simulink model "sim_impcont"  (R2016a)
settings: Solver=ode23tb  StartTime=0.0  StopTime=t(end)  MaxStep=1e-3
InitFcn:
  | fp_k=12000;
  | fp_d=10*2e2;
  | w=11;
  | stiff=0.1;
  | damp=1;
values from neighbouring files (symbols this model uses):
  N = length(shin_angles_in.signals.values)    [GaitEmu_code.m]    (also in dy1.m; dy2.m; est_joint.m = size( [body1.trans body2.trans], 1 ); impcont.m)
  s = [-atan((t2.*3.379e-4+t3+t4.*t5.*4.401e-2)./(t4.*cos(q2)));-asin(t2.*1.4870979e-5+t3.*4.401e-2-t4.*t5)]    [FK_af.m]    (also in FK_footimp.m = [atan((ree2_1.*t2.*4.401e-2+ree2_2.*t4+ree2_3.*t3+t5.*t7.*4.; FK_gaitEmul.m = [q1+t2.*t4.*4.234e-1+t3.*t5.*1.5e-3-t2.*t6.*t7.*1.5e-3-5.347; ik.m = [x; y; z]; ik_af.m = FK_af(q))
  sta = [-0.5345 0.03779 -0.0866]    [GaitEmu_code.m]    (also in dy1.m; dy2.m; grn_dyn.m; impcont.m)
  Y = -( reshape( body1.trans', [], 1 ) - reshape( body2.trans', [], 1 ) )    [creat_joint.m]    (also in est_joint.m = -( reshape( body1.trans', [3*N 1] ) - reshape( body2.trans',)
undefined symbols (not defined in the file or in its folder): X, Z
libraries: sm_lib x261, nesl_utility x84, simulink x3, dspstat3 x1
(part 1 of 6)
settings Model: Creator=lcasteli  LastModifiedBy=lcasteli
settings SolverCC: ZeroCrossControl=DisableAll
settings DataIOCC: OutputTimes=[0:0.01:t(end)]

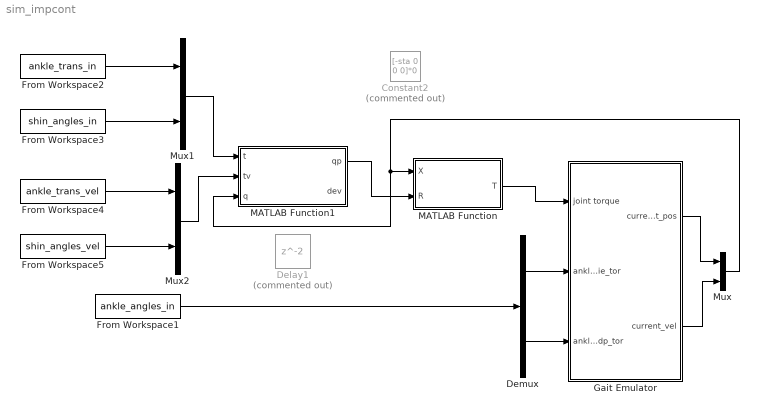
== system sim_impcont ==
  Constant2 : Constant  Commented=on  Value=[-sta 0 0 0]*0
  Delay1 : Delay  Commented=on  SampleTime=0.01
  Demux : Demux  Outputs=2
  From Workspace1 : FromWorkspace  VariableName=ankle_angles_in  SampleTime=0
  From Workspace2 : FromWorkspace  VariableName=ankle_trans_in  SampleTime=0
  From Workspace3 : FromWorkspace  VariableName=shin_angles_in  SampleTime=0
  From Workspace4 : FromWorkspace  VariableName=ankle_trans_vel  SampleTime=0
  From Workspace5 : FromWorkspace  VariableName=shin_angles_vel  SampleTime=0
  Gait Emulator : Subsystem
  MATLAB Function : MATLAB Function  TreatAsAtomicUnit=on
  MATLAB Function1 : MATLAB Function  TreatAsAtomicUnit=on
  Mux : Mux  Inputs=2
  Mux1 : Mux  Inputs=2
  Mux2 : Mux  Inputs=2
  wires:
  Demux/1 -> Gait Emulator/2(ankle_ie_tor)
  Demux/2 -> Gait Emulator/3(ankle_dp_tor)
  From Workspace1/1 -> Demux/1
  Mux1/1 -> MATLAB Function1/1(t)
  From Workspace2/1 -> Mux1/1
  From Workspace3/1 -> Mux1/2
  MATLAB Function1/1(qp) -> MATLAB Function/2(R)
  Gait Emulator/1(current_pos) -> Mux/1
  Gait Emulator/2(current_vel) -> Mux/2
  Mux/1 -> MATLAB Function1/3(q), MATLAB Function/1(X)
  MATLAB Function/1(T) -> Gait Emulator/1(joint torque)
  From Workspace4/1 -> Mux2/1
  From Workspace5/1 -> Mux2/2
  Mux2/1 -> MATLAB Function1/2(tv)

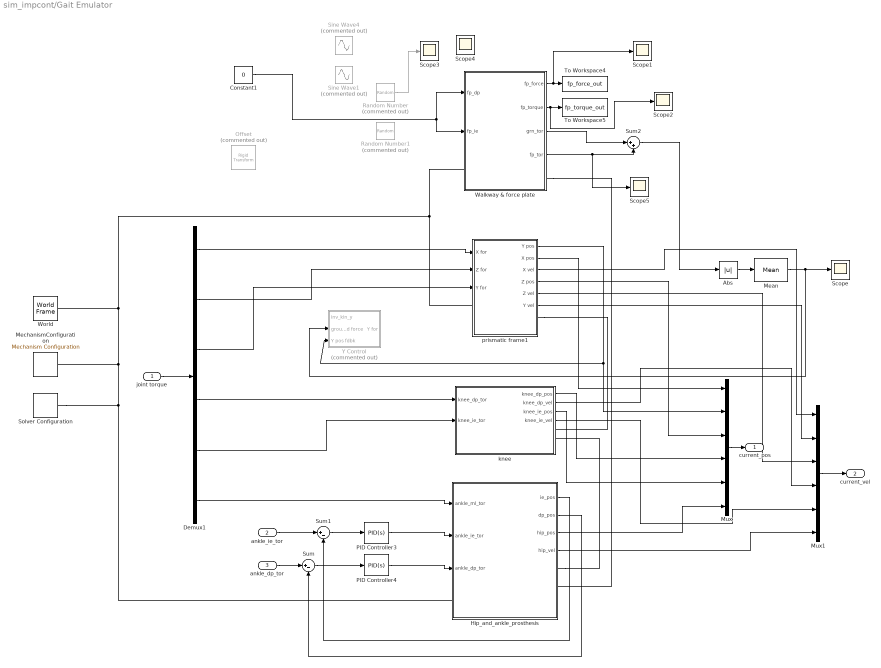
== system sim_impcont/Gait Emulator ==
  joint torque : Inport
  ankle_ie_tor : Inport  Port=2
  ankle_dp_tor : Inport  Port=3
  Abs : Abs
  Constant1 : Constant  Value=0
  Demux1 : Demux  Outputs=6
  Hip_and_ankle_prosthesis : Subsystem
  Mean : dspstat3/Mean  run=off  reset_popup=None  InputProcessing=Columns as channels (frame based)  directionMode=Each column  dimension=1  roiEnable=off  roiType=Rectangles  roiPortion=Entire ROI  roiOutput=Individual statistics for each ROI  roiFlag=off  outputDataTypeStr=Inherit: Same as accumulator  outputLastDataTypeStr=Inherit: Same as accumulator  outputMin=[]  outputMax=[]  roundingMode=Floor  overflowMode=off
  MechanismConfiguration : sm_lib/Utilities/Mechanism Configuration  UniformGravity=Constant  GravityVector=[0 -9.81 0]  GravityUnits=m/s^2  LinearizationDelta=0.001
  Mux : Mux  Inputs=6
  Mux1 : Mux  Inputs=6
  Offset : sm_lib/Frames and Transforms/Rigid Transform  Commented=on  TranslationMethod=Cartesian  TranslationLengthUnit=m  TranslationStandardAxis=+Z  TranslationStandardOffset=0  TranslationCartesianOffset=[0.5345 0 -0.03779]  TranslationROffset=0  TranslationROffsetUnits=m  TranslationZOffset=0  TranslationZOffsetUnits=m  TranslationThetaOffset=0  TranslationThetaOffsetUnits=deg  RotationMethod=None  RotationAngleUnits=deg  RotationStandardAxis=+Z  RotationAngle=0.0  RotationArbitraryAxis=[0 0 1]  FollAlignAxisA=+X  BaseAlignAxisA=+Y  FollAlignAxisB=+Y  BaseAlignAxisB=+Z  RotationSequenceAxes=FollowerAxes  RotationSequence=XYX  RotationSequenceAngles=[0 0 0]  RotationSequenceAnglesUnits=deg  RotationMatrix=[1 0 0; 0 1 0; 0 0 1]
  PID Controller3 : simulink/Continuous/PID Controller  Controller=PID  TimeDomain=Continuous-time  SampleTime=-1  IntegratorMethod=Forward Euler  FilterMethod=Forward Euler  Form=Parallel  UseFilter=on  ControllerParametersSource=internal  P=107.335597273016  I=2166.16665425047  D=0.120593585905197  N=113.306431529722  InitialConditionSource=internal  InitialConditionForIntegrator=0  InitialConditionForFilter=0  ExternalReset=none  LimitOutput=on  UpperSaturationLimit=300  LowerSaturationLimit=-300  LinearizeAsGain=on  AntiWindupMode=clamping  Kb=1  TrackingMode=off  Kt=1  PParamMin=[]  PParamMax=[]  IParamMin=[]  IParamMax=[]  DParamMin=[]  DParamMax=[]  NParamMin=[]  NParamMax=[]  KbParamMin=[]  KbParamMax=[]  KtParamMin=[]  KtParamMax=[]  POutMin=[]  POutMax=[]  IOutMin=[]  IOutMax=[]  DOutMin=[]  DOutMax=[]  NOutMin=[]  NOutMax=[]  KbOutMin=[]  KbOutMax=[]  KtOutMin=[]  KtOutMax=[]  IntegratorOutMin=[]  IntegratorOutMax=[]  FilterOutMin=[]  FilterOutMax=[]  SumOutMin=[]  SumOutMax=[]  SumI1OutMin=[]  SumI1OutMax=[]  SumI2OutMin=[]  SumI2OutMax=[]  SumI3OutMin=[]  SumI3OutMax=[]  SumDOutMin=[]  SumDOutMax=[]  SaturationOutMin=[]  SaturationOutMax=[]  IntegratorContinuousStateAttributes=''  IntegratorStateMustResolveToSignalObject=off  IntegratorRTWStateStorageClass=Auto  FilterContinuousStateAttributes=''  FilterStateMustResolveToSignalObject=off  FilterRTWStateStorageClass=Auto  DifferentiatorICPrevScaledInput=0  DifferentiatorOutMin=[]  DifferentiatorOutMax=[]
  PID Controller4 : simulink/Continuous/PID Controller  Controller=PID  TimeDomain=Continuous-time  SampleTime=-1  IntegratorMethod=Forward Euler  FilterMethod=Forward Euler  Form=Parallel  UseFilter=on  ControllerParametersSource=internal  P=105.568672508167  I=2116.13308642224  D=0.177175601648911  N=114.243233016109  InitialConditionSource=internal  InitialConditionForIntegrator=0  InitialConditionForFilter=0  ExternalReset=none  LimitOutput=on  UpperSaturationLimit=300  LowerSaturationLimit=-300  LinearizeAsGain=on  AntiWindupMode=clamping  Kb=1  TrackingMode=off  Kt=1  PParamMin=[]  PParamMax=[]  IParamMin=[]  IParamMax=[]  DParamMin=[]  DParamMax=[]  NParamMin=[]  NParamMax=[]  KbParamMin=[]  KbParamMax=[]  KtParamMin=[]  KtParamMax=[]  POutMin=[]  POutMax=[]  IOutMin=[]  IOutMax=[]  DOutMin=[]  DOutMax=[]  NOutMin=[]  NOutMax=[]  KbOutMin=[]  KbOutMax=[]  KtOutMin=[]  KtOutMax=[]  IntegratorOutMin=[]  IntegratorOutMax=[]  FilterOutMin=[]  FilterOutMax=[]  SumOutMin=[]  SumOutMax=[]  SumI1OutMin=[]  SumI1OutMax=[]  SumI2OutMin=[]  SumI2OutMax=[]  SumI3OutMin=[]  SumI3OutMax=[]  SumDOutMin=[]  SumDOutMax=[]  SaturationOutMin=[]  SaturationOutMax=[]  IntegratorContinuousStateAttributes=''  IntegratorStateMustResolveToSignalObject=off  IntegratorRTWStateStorageClass=Auto  FilterContinuousStateAttributes=''  FilterStateMustResolveToSignalObject=off  FilterRTWStateStorageClass=Auto  DifferentiatorICPrevScaledInput=0  DifferentiatorOutMin=[]  DifferentiatorOutMax=[]
  Random Number : RandomNumber  Commented=on  Variance=1e4  SampleTime=0.1
  Random Number1 : RandomNumber  Commented=on  Variance=4e3  SampleTime=0.1
  Scope{,1..5} (6 alike) : Scope
  Sine Wave1 : Sin  Commented=on  Amplitude=100  Frequency=10  Phase=pi/6  SampleTime=0.001
  Sine Wave4 : Sin  Commented=on  Amplitude=100*2  Frequency=10  SampleTime=0.001
  Solver Configuration : nesl_utility/Solver Configuration  PhysicalDomain=network_engine_domain  SubClassName=solver  LeftPortType=input  RightPortType=generic  Accelerate=off  Tones=[]  Harmonics=[]  SimulateNoise=off  Profile=off  UseLocalSampling=off  EnableSwitchedLinearOptims=on  FrequencyDomain=off  UseCCode=off  RelTol=0.001  AbsTol=1e-06  MinStep=1e-09  ToWorkspace=off  RevertToSquareIcSolve=off  NumHomotopyIterations=100  PhasorMode=off  PhasorModeNumHarmonics=1  OverrideAbsTol=off  DoDC=off  ResidualTolerance=1e-09  UseLocalSolver=off  LocalSolverChoice=NE_BACKWARD_EULER_ADVANCER  LocalSolverSampleTime=0.001  DoFixedCost=off  MaxNonlinIter=3  MaxModeIter=2  LinearAlgebra=Sparse  DelaysMemoryBudget=1024  AutomaticFiltering=on  FilteringTimeConstant=0.001
  Sum : Sum  Inputs=|+-
  Sum1 : Sum  Inputs=|+-
  Sum2 : Sum  Inputs=|++
  To Workspace4 : ToWorkspace  VariableName=fp_force_out  SaveFormat=Structure With Time  SampleTime=-1
  To Workspace5 : ToWorkspace  VariableName=fp_torque_out  SaveFormat=Structure With Time  SampleTime=-1
  Walkway & force plate : Subsystem
  World : sm_lib/Frames and Transforms/World Frame
  Y Control : Subsystem  Commented=on
  "knee " : Subsystem
  prismatic frame1 : Subsystem
  current_pos : Outport
  current_vel : Outport  Port=2
  wires:
  joint torque/1 -> Demux1/1
  Walkway & force plate/2(fp_torque) -> Scope2/1, To Workspace5/1
  Walkway & force plate/1(fp_force) -> Scope1/1, To Workspace4/1
  Demux1/4 -> "knee "/1(knee_dp_tor)
  Demux1/5 -> "knee "/2(knee_ie_tor)
  Demux1/6 -> Hip_and_ankle_prosthesis/1(ankle_ml_tor)
  Walkway & force plate/3(grn_tor) -> Sum2/1
  Walkway & force plate/4(fp_tor) -> Scope5/1, Sum2/2
  Sum2/1 -> Abs/1
  Abs/1 -> Mean/1
  Mean/1 -> Y Control/2(ground force), Scope/1
  ankle_ie_tor/1 -> Sum1/1
  ankle_dp_tor/1 -> Sum/1
  Hip_and_ankle_prosthesis/2(dp_pos) -> Sum/2
  Hip_and_ankle_prosthesis/1(ie_pos) -> Sum1/2
  PID Controller4/1 -> Hip_and_ankle_prosthesis/3(ankle_dp_tor)
  PID Controller3/1 -> Hip_and_ankle_prosthesis/2(ankle_ie_tor)
  Sum1/1 -> PID Controller3/1
  Sum/1 -> PID Controller4/1
  Random Number/1 -> Scope3/1
  Constant1/1 -> Walkway & force plate/1(fp_dp), Walkway & force plate/2(fp_ie)
  prismatic frame1/1(Y pos) -> Mux/2, Y Control/3(Y pos fdbk)
  Demux1/1 -> prismatic frame1/1(X for)
  Demux1/2 -> prismatic frame1/2(Z for)
  prismatic frame1/2(X pos) -> Mux/1
  prismatic frame1/4(Z pos) -> Mux/3
  prismatic frame1/3(X vel) -> Mux1/1
  prismatic frame1/6(Y vel) -> Mux1/2
  prismatic frame1/5(Z vel) -> Mux1/3
  "knee "/1(knee_dp_pos) -> Mux/4
  "knee "/3(knee_ie_pos) -> Mux/5
  "knee "/4(knee_ie_vel) -> Mux1/5
  "knee "/2(knee_dp_vel) -> Mux1/4
  Hip_and_ankle_prosthesis/3(hip_pos) -> Mux/6
  Hip_and_ankle_prosthesis/4(hip_vel) -> Mux1/6
  Mux1/1 -> current_vel/1
  Mux/1 -> current_pos/1
  Demux1/3 -> prismatic frame1/3(Y for)
  connections:
  Hip_and_ankle_prosthesis/RConn1 -- "knee "/RConn2
  Walkway & force plate/RConn1 -- Hip_and_ankle_prosthesis/RConn2
  Walkway & force plate/LConn1 -- prismatic frame1/LConn1 -- Hip_and_ankle_prosthesis/LConn1 -- Solver Configuration/RConn1 -- MechanismConfiguration/RConn1 -- World/RConn1
  prismatic frame1/RConn1 -- "knee "/RConn1

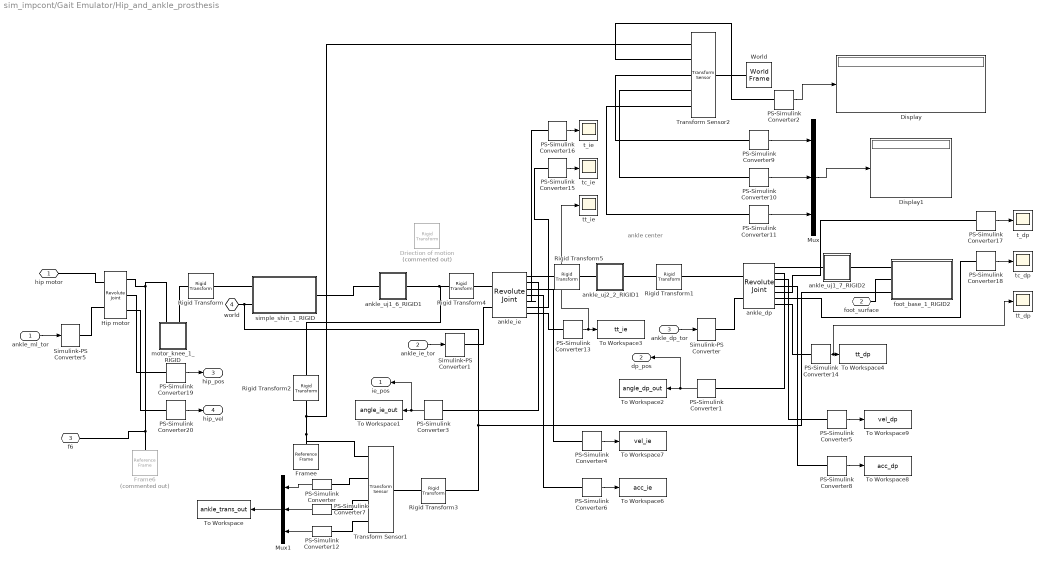
== system sim_impcont/Gait Emulator/Hip_and_ankle_prosthesis ==
  note: ankle center
  ankle_ml_tor : Inport
  ankle_ie_tor : Inport  Port=2
  ankle_dp_tor : Inport  Port=3
  Display : Display
  Display1 : Display
  Driection of motion : sm_lib/Frames and Transforms/Rigid Transform  Commented=on  TranslationMethod=None  TranslationLengthUnit=m  TranslationStandardAxis=+Z  TranslationStandardOffset=0  TranslationCartesianOffset=[0 0 0]  TranslationROffset=0  TranslationROffsetUnits=m  TranslationZOffset=0  TranslationZOffsetUnits=m  TranslationThetaOffset=0  TranslationThetaOffsetUnits=deg  RotationMethod=StandardAxis  RotationAngleUnits=deg  RotationStandardAxis=+Z  RotationAngle=0  RotationArbitraryAxis=[0 0 1]  FollAlignAxisA=+X  BaseAlignAxisA=+Y  FollAlignAxisB=+Y  BaseAlignAxisB=+Z  RotationSequenceAxes=FollowerAxes  RotationSequence=XYX  RotationSequenceAngles=[0 0 0]  RotationSequenceAnglesUnits=deg  RotationMatrix=[1 0 0; 0 1 0; 0 0 1]
  Frame6 : sm_lib/Frames and Transforms/Reference Frame  Commented=on
  Framee : sm_lib/Frames and Transforms/Reference Frame
  Hip motor : sm_lib/Joints/Revolute Joint  SenseConstraintForce=off  SenseConstraintForceX=off  SenseConstraintForceY=off  SenseConstraintForceZ=off  SenseConstraintTorque=off  SenseConstraintTorqueX=off  SenseConstraintTorqueY=off  SenseConstraintTorqueZ=off  SenseTotalForce=off  SenseTotalForceX=off  SenseTotalForceY=off  SenseTotalForceZ=off  SenseTotalTorque=off  SenseTotalTorqueX=off  SenseTotalTorqueY=off  SenseTotalTorqueZ=off  CompositeWrenchDir=FollowerOnBase  CompositeWrenchFrame=BaseFrame  EquilibriumPosition=0  EquilibriumPositionUnits=rad  SpringStiffness=stiff  SpringStiffnessUnits=m*N/rad  DampingCoefficient=damp  DampingCoefficientUnits=m*s*N/rad  TorqueActuationMode=InputTorque  MotionActuationMode=ComputedMotion  SensePosition=on  SenseVelocity=on  SenseAcceleration=off  SenseTorqueForce=off  PositionTargetSpecify=off  PositionTargetPriority=Low  PositionTargetValue=0  PositionTargetValueUnits=deg  VelocityTargetSpecify=off  VelocityTargetPriority=High  VelocityTargetValue=0  VelocityTargetValueUnits=deg/s
  Mux : Mux  Inputs=3
  Mux1 : Mux  Inputs=3
  PS-Simulink Converter{,1..20} (21 alike) : nesl_utility/PS-Simulink Converter  PhysicalDomain=network_engine_domain  SubClassName=ps_output  LeftPortType=input  RightPortType=output  PseudoPeriodic=off  Frequencies=[]  Unit=1  AffineConversion=off
  Rigid Transform : sm_lib/Frames and Transforms/Rigid Transform  TranslationMethod=StandardAxis  TranslationLengthUnit=m  TranslationStandardAxis=+Z  TranslationStandardOffset=0.15  TranslationCartesianOffset=[0 0 0]  TranslationROffset=0  TranslationROffsetUnits=m  TranslationZOffset=0  TranslationZOffsetUnits=m  TranslationThetaOffset=0  TranslationThetaOffsetUnits=deg  RotationMethod=StandardAxis  RotationAngleUnits=deg  RotationStandardAxis=+X  RotationAngle=180  RotationArbitraryAxis=[1 0 1]  FollAlignAxisA=+X  BaseAlignAxisA=+Y  FollAlignAxisB=+Y  BaseAlignAxisB=+Z  RotationSequenceAxes=FollowerAxes  RotationSequence=XYX  RotationSequenceAngles=[0 0 0]  RotationSequenceAnglesUnits=deg  RotationMatrix=[1 0 0; 0 1 0; 0 0 1]
  Rigid Transform1 : sm_lib/Frames and Transforms/Rigid Transform  TranslationMethod=None  TranslationLengthUnit=m  TranslationStandardAxis=+Z  TranslationStandardOffset=0.15  TranslationCartesianOffset=[0 0 0]  TranslationROffset=0  TranslationROffsetUnits=m  TranslationZOffset=0  TranslationZOffsetUnits=m  TranslationThetaOffset=0  TranslationThetaOffsetUnits=deg  RotationMethod=StandardAxis  RotationAngleUnits=deg  RotationStandardAxis=+Z  RotationAngle=-90  RotationArbitraryAxis=[1 0 1]  FollAlignAxisA=+X  BaseAlignAxisA=+Y  FollAlignAxisB=+Y  BaseAlignAxisB=+Z  RotationSequenceAxes=FollowerAxes  RotationSequence=XYX  RotationSequenceAngles=[0 0 0]  RotationSequenceAnglesUnits=deg  RotationMatrix=[1 0 0; 0 1 0; 0 0 1]
  Rigid Transform2 : sm_lib/Frames and Transforms/Rigid Transform  TranslationMethod=StandardAxis  TranslationLengthUnit=m  TranslationStandardAxis=+Z  TranslationStandardOffset=-8.5e-3  TranslationCartesianOffset=[0 0 0]  TranslationROffset=0  TranslationROffsetUnits=m  TranslationZOffset=0  TranslationZOffsetUnits=m  TranslationThetaOffset=0  TranslationThetaOffsetUnits=deg  RotationMethod=AlignedAxes  RotationAngleUnits=deg  RotationStandardAxis=+Z  RotationAngle=-90  RotationArbitraryAxis=[1 0 1]  FollAlignAxisA=+X  BaseAlignAxisA=-Z  FollAlignAxisB=+Y  BaseAlignAxisB=-Y  RotationSequenceAxes=FollowerAxes  RotationSequence=XYX  RotationSequenceAngles=[0 0 0]  RotationSequenceAnglesUnits=deg  RotationMatrix=[1 0 0; 0 1 0; 0 0 1]
  Rigid Transform3 : sm_lib/Frames and Transforms/Rigid Transform  TranslationMethod=StandardAxis  TranslationLengthUnit=m  TranslationStandardAxis=+Y  TranslationStandardOffset=0.1517  TranslationCartesianOffset=[0 0 0]  TranslationROffset=0  TranslationROffsetUnits=m  TranslationZOffset=0  TranslationZOffsetUnits=m  TranslationThetaOffset=0  TranslationThetaOffsetUnits=deg  RotationMethod=None  RotationAngleUnits=deg  RotationStandardAxis=+Z  RotationAngle=0.0  RotationArbitraryAxis=[0 0 1]  FollAlignAxisA=+X  BaseAlignAxisA=+Y  FollAlignAxisB=+Y  BaseAlignAxisB=+Z  RotationSequenceAxes=FollowerAxes  RotationSequence=XYX  RotationSequenceAngles=[0 0 0]  RotationSequenceAnglesUnits=deg  RotationMatrix=[1 0 0; 0 1 0; 0 0 1]
  Rigid Transform4 : sm_lib/Frames and Transforms/Rigid Transform  TranslationMethod=StandardAxis  TranslationLengthUnit=m  TranslationStandardAxis=+Z  TranslationStandardOffset=-8.5e-3  TranslationCartesianOffset=[0 0 0]  TranslationROffset=0  TranslationROffsetUnits=m  TranslationZOffset=0  TranslationZOffsetUnits=m  TranslationThetaOffset=0  TranslationThetaOffsetUnits=deg  RotationMethod=None  RotationAngleUnits=deg  RotationStandardAxis=+Z  RotationAngle=0.0  RotationArbitraryAxis=[0 0 1]  FollAlignAxisA=+X  BaseAlignAxisA=+Y  FollAlignAxisB=+Y  BaseAlignAxisB=+Z  RotationSequenceAxes=FollowerAxes  RotationSequence=XYX  RotationSequenceAngles=[0 0 0]  RotationSequenceAnglesUnits=deg  RotationMatrix=[1 0 0; 0 1 0; 0 0 1]
  Rigid Transform5 : sm_lib/Frames and Transforms/Rigid Transform  TranslationMethod=StandardAxis  TranslationLengthUnit=m  TranslationStandardAxis=+Z  TranslationStandardOffset=8.5e-3  TranslationCartesianOffset=[0 0 0]  TranslationROffset=0  TranslationROffsetUnits=m  TranslationZOffset=0  TranslationZOffsetUnits=m  TranslationThetaOffset=0  TranslationThetaOffsetUnits=deg  RotationMethod=None  RotationAngleUnits=deg  RotationStandardAxis=+Z  RotationAngle=0.0  RotationArbitraryAxis=[0 0 1]  FollAlignAxisA=+X  BaseAlignAxisA=+Y  FollAlignAxisB=+Y  BaseAlignAxisB=+Z  RotationSequenceAxes=FollowerAxes  RotationSequence=XYX  RotationSequenceAngles=[0 0 0]  RotationSequenceAnglesUnits=deg  RotationMatrix=[1 0 0; 0 1 0; 0 0 1]
  Simulink-PS Converter : nesl_utility/Simulink-PS Converter  PhysicalDomain=network_engine_domain  SubClassName=ps_input  LeftPortType=input  RightPortType=output  PseudoPeriodic=off  Frequencies=[]  NoiseDistribution=none  NoiseParameters=[]  Unit=1  AffineConversion=off  InputFiltering=on  SimscapeFilterOrder=2  InputFilterTimeConstant=0.001  UdotUserProvided=1
  Simulink-PS Converter1 : nesl_utility/Simulink-PS Converter  PhysicalDomain=network_engine_domain  SubClassName=ps_input  LeftPortType=input  RightPortType=output  PseudoPeriodic=off  Frequencies=[]  NoiseDistribution=none  NoiseParameters=[]  Unit=1  AffineConversion=off  InputFiltering=on  SimscapeFilterOrder=2  InputFilterTimeConstant=0.001  UdotUserProvided=2
  Simulink-PS Converter5 : nesl_utility/Simulink-PS Converter  PhysicalDomain=network_engine_domain  SubClassName=ps_input  LeftPortType=input  RightPortType=output  PseudoPeriodic=off  Frequencies=[]  NoiseDistribution=none  NoiseParameters=[]  Unit=1  AffineConversion=off  InputFiltering=on  SimscapeFilterOrder=2  InputFilterTimeConstant=0.001  UdotUserProvided=2
  To Workspace : ToWorkspace  VariableName=ankle_trans_out  SaveFormat=Structure With Time  SampleTime=-1
  To Workspace1 : ToWorkspace  VariableName=angle_ie_out  SaveFormat=Structure With Time  SampleTime=-1
  To Workspace2 : ToWorkspace  VariableName=angle_dp_out  SaveFormat=Structure With Time  SampleTime=-1
  To Workspace3 : ToWorkspace  VariableName=tt_ie  SaveFormat=Structure With Time  SampleTime=-1
  To Workspace4 : ToWorkspace  VariableName=tt_dp  SaveFormat=Structure With Time  SampleTime=-1
  To Workspace6 : ToWorkspace  VariableName=acc_ie  SaveFormat=Structure With Time  SampleTime=-1
  To Workspace7 : ToWorkspace  VariableName=vel_ie  SaveFormat=Structure With Time  SampleTime=-1
  To Workspace8 : ToWorkspace  VariableName=acc_dp  SaveFormat=Structure With Time  SampleTime=-1
  To Workspace9 : ToWorkspace  VariableName=vel_dp  SaveFormat=Structure With Time  SampleTime=-1
  Transform Sensor1 : sm_lib/Frames and Transforms/Transform Sensor  MeasurementFrame=Base  SenseAngle=off  SenseAxis=off  SenseAngle1=off  SenseAngle2=off  SenseAngle3=off  SenseQ=off  SenseR=off  SenseOmegaX=off  SenseOmegaY=off  SenseOmegaZ=off  SenseOmega1=off  SenseOmega2=off  SenseOmega3=off  SenseQDot=off  SenseRDot=off  SenseAlphaX=off  SenseAlphaY=off  SenseAlphaZ=off  SenseAlpha1=off  SenseAlpha2=off  SenseAlpha3=off  SenseQDDot=off  SenseRDDot=off  SenseX=on  SenseY=on  SenseZ=on  SenseRad=off  SenseAzim=off  SenseDist=off  SenseInc=off  SenseXDot=off  SenseYDot=off  SenseZDot=off  SenseRadDot=off  SenseAzimDot=off  SenseDistDot=off  SenseIncDot=off  SenseXDDot=off  SenseYDDot=off  SenseZDDot=off  SenseRadDDot=off  SenseAzimDDot=off  SenseDistDDot=off  SenseIncDDot=off
  Transform Sensor2 : sm_lib/Frames and Transforms/Transform Sensor  MeasurementFrame=Base  SenseAngle=off  SenseAxis=off  SenseAngle1=off  SenseAngle2=off  SenseAngle3=off  SenseQ=off  SenseR=on  SenseOmegaX=off  SenseOmegaY=off  SenseOmegaZ=off  SenseOmega1=off  SenseOmega2=off  SenseOmega3=off  SenseQDot=off  SenseRDot=off  SenseAlphaX=off  SenseAlphaY=off  SenseAlphaZ=off  SenseAlpha1=off  SenseAlpha2=off  SenseAlpha3=off  SenseQDDot=off  SenseRDDot=off  SenseX=on  SenseY=on  SenseZ=on  SenseRad=off  SenseAzim=off  SenseDist=off  SenseInc=off  SenseXDot=off  SenseYDot=off  SenseZDot=off  SenseRadDot=off  SenseAzimDot=off  SenseDistDot=off  SenseIncDot=off  SenseXDDot=off  SenseYDDot=off  SenseZDDot=off  SenseRadDDot=off  SenseAzimDDot=off  SenseDistDDot=off  SenseIncDDot=off
  World : sm_lib/Frames and Transforms/World Frame
  ankle_dp : sm_lib/Joints/Revolute Joint  SenseConstraintForce=off  SenseConstraintForceX=off  SenseConstraintForceY=off  SenseConstraintForceZ=off  SenseConstraintTorque=on  SenseConstraintTorqueX=off  SenseConstraintTorqueY=off  SenseConstraintTorqueZ=off  SenseTotalForce=off  SenseTotalForceX=off  SenseTotalForceY=off  SenseTotalForceZ=off  SenseTotalTorque=on  SenseTotalTorqueX=off  SenseTotalTorqueY=off  SenseTotalTorqueZ=off  CompositeWrenchDir=FollowerOnBase  CompositeWrenchFrame=BaseFrame  EquilibriumPosition=0  EquilibriumPositionUnits=rad  SpringStiffness=stiff_dp  SpringStiffnessUnits=m*N/rad  DampingCoefficient=damp_dp  DampingCoefficientUnits=m*s*N/rad  TorqueActuationMode=InputTorque  MotionActuationMode=ComputedMotion  SensePosition=on  SenseVelocity=on  SenseAcceleration=on  SenseTorqueForce=on  PositionTargetSpecify=off  PositionTargetPriority=Low  PositionTargetValue=-90  PositionTargetValueUnits=deg  VelocityTargetSpecify=off  VelocityTargetPriority=High  VelocityTargetValue=0  VelocityTargetValueUnits=deg/s
  ankle_ie : sm_lib/Joints/Revolute Joint  SenseConstraintForce=off  SenseConstraintForceX=off  SenseConstraintForceY=off  SenseConstraintForceZ=off  SenseConstraintTorque=on  SenseConstraintTorqueX=off  SenseConstraintTorqueY=off  SenseConstraintTorqueZ=off  SenseTotalForce=off  SenseTotalForceX=off  SenseTotalForceY=off  SenseTotalForceZ=off  SenseTotalTorque=on  SenseTotalTorqueX=off  SenseTotalTorqueY=off  SenseTotalTorqueZ=off  CompositeWrenchDir=FollowerOnBase  CompositeWrenchFrame=BaseFrame  EquilibriumPosition=0  EquilibriumPositionUnits=rad  SpringStiffness=stiff_ie  SpringStiffnessUnits=N*m/rad  DampingCoefficient=damp_ie  DampingCoefficientUnits=m*s*N/rad  TorqueActuationMode=InputTorque  MotionActuationMode=ComputedMotion  SensePosition=on  SenseVelocity=on  SenseAcceleration=on  SenseTorqueForce=on  PositionTargetSpecify=off  PositionTargetPriority=Low  PositionTargetValue=0  PositionTargetValueUnits=deg  VelocityTargetSpecify=off  VelocityTargetPriority=High  VelocityTargetValue=0  VelocityTargetValueUnits=deg/s
  ankle_uj1_6_RIGID1 : Subsystem
  ankle_uj1_7_RIGID2 : Subsystem
  ankle_uj2_2_RIGID1 : Subsystem
  foot_base_1_RIGID2 : Subsystem
  motor_knee_1_RIGID : Subsystem
  simple_shin_1_RIGID : Subsystem
  t_dp : Scope
  t_ie : Scope
  tc_dp : Scope
  tc_ie : Scope
  tt_dp : Scope
  tt_ie : Scope
  hip motor : PMIOPort  Port=1  Side=Right
  foot_surface : PMIOPort  Port=2  Side=Right
  f6 : PMIOPort  Port=3  Side=Right
  world : PMIOPort  Port=4  Side=Left
  ie_pos : Outport
  dp_pos : Outport  Port=2
  hip_pos : Outport  Port=3
  hip_vel : Outport  Port=4
  wires:
  PS-Simulink Converter1/1 -> dp_pos/1, To Workspace2/1
  PS-Simulink Converter4/1 -> To Workspace7/1
  PS-Simulink Converter5/1 -> To Workspace9/1
  PS-Simulink Converter6/1 -> To Workspace6/1
  PS-Simulink Converter8/1 -> To Workspace8/1
  PS-Simulink Converter9/1 -> Mux/1
  PS-Simulink Converter10/1 -> Mux/2
  PS-Simulink Converter11/1 -> Mux/3
  Mux/1 -> Display1/1
  ankle_ml_tor/1 -> Simulink-PS Converter5/1
  PS-Simulink Converter2/1 -> Display/1
  PS-Simulink Converter3/1 -> ie_pos/1, To Workspace1/1
  ankle_dp_tor/1 -> Simulink-PS Converter/1
  PS-Simulink Converter/1 -> Mux1/1
  PS-Simulink Converter7/1 -> Mux1/2
  PS-Simulink Converter12/1 -> Mux1/3
  Mux1/1 -> To Workspace/1
  PS-Simulink Converter13/1 -> tt_ie/1, To Workspace3/1
  PS-Simulink Converter14/1 -> tt_dp/1, To Workspace4/1
  PS-Simulink Converter18/1 -> tc_dp/1
  PS-Simulink Converter17/1 -> t_dp/1
  PS-Simulink Converter15/1 -> tc_ie/1
  PS-Simulink Converter16/1 -> t_ie/1
  ankle_ie_tor/1 -> Simulink-PS Converter1/1
  PS-Simulink Converter19/1 -> hip_pos/1
  PS-Simulink Converter20/1 -> hip_vel/1
  connections:
  ankle_uj2_2_RIGID1/LConn1 -- Rigid Transform5/RConn1
  Rigid Transform1/RConn1 -- ankle_dp/LConn1
  simple_shin_1_RIGID/LConn1 -- Rigid Transform/RConn1
  Rigid Transform/LConn1 -- motor_knee_1_RIGID/RConn2
  ankle_uj2_2_RIGID1/RConn1 -- Rigid Transform1/LConn1
  Hip motor/RConn1 -- motor_knee_1_RIGID/RConn1 -- Frame6/RConn1 -- f6/RConn1
  Hip motor/LConn1 -- hip motor/RConn1
  PS-Simulink Converter4/LConn1 -- ankle_ie/RConn3
  PS-Simulink Converter5/LConn1 -- ankle_dp/RConn3
  PS-Simulink Converter6/LConn1 -- ankle_ie/RConn4
  PS-Simulink Converter8/LConn1 -- ankle_dp/RConn4
  foot_base_1_RIGID2/LConn1 -- ankle_uj1_7_RIGID2/RConn1
  ankle_uj1_7_RIGID2/LConn1 -- ankle_dp/RConn1
  foot_base_1_RIGID2/LConn2 -- foot_surface/RConn1
  PS-Simulink Converter3/LConn1 -- ankle_ie/RConn2
  PS-Simulink Converter1/LConn1 -- ankle_dp/RConn2
  Transform Sensor2/LConn1 -- World/RConn1
  Transform Sensor2/RConn2 -- PS-Simulink Converter2/LConn1
  Transform Sensor2/RConn3 -- PS-Simulink Converter9/LConn1
  Transform Sensor2/RConn4 -- PS-Simulink Converter10/LConn1
  Transform Sensor2/RConn5 -- PS-Simulink Converter11/LConn1
  Framee/RConn1 -- Rigid Transform2/RConn1 -- Transform Sensor2/RConn1 -- Transform Sensor1/RConn1
  simple_shin_1_RIGID/RConn1 -- ankle_uj1_6_RIGID1/LConn1
  Rigid Transform3/RConn1 -- Transform Sensor1/LConn1
  Transform Sensor1/RConn2 -- PS-Simulink Converter/LConn1
  Transform Sensor1/RConn3 -- PS-Simulink Converter7/LConn1
  Transform Sensor1/RConn4 -- PS-Simulink Converter12/LConn1
  ankle_ie/RConn6 -- PS-Simulink Converter15/LConn1
  ankle_ie/RConn7 -- PS-Simulink Converter13/LConn1
  ankle_ie/RConn5 -- PS-Simulink Converter16/LConn1
  ankle_dp/RConn7 -- PS-Simulink Converter14/LConn1
  ankle_dp/RConn5 -- PS-Simulink Converter17/LConn1
  ankle_dp/RConn6 -- PS-Simulink Converter18/LConn1
  Rigid Transform2/LConn1 -- ankle_uj1_6_RIGID1/RConn1 -- Rigid Transform4/LConn1
  Rigid Transform4/RConn1 -- ankle_ie/LConn1
  Rigid Transform5/LConn1 -- ankle_ie/RConn1
  ankle_dp/LConn2 -- Simulink-PS Converter/RConn1
  world/RConn1 -- Rigid Transform3/LConn1 -- foot_base_1_RIGID2/LConn3 -- simple_shin_1_RIGID/LConn2
  Simulink-PS Converter5/RConn1 -- Hip motor/LConn2
  ankle_ie/LConn2 -- Simulink-PS Converter1/RConn1
  Hip motor/RConn2 -- PS-Simulink Converter19/LConn1
  Hip motor/RConn3 -- PS-Simulink Converter20/LConn1

== system sim_impcont/Gait Emulator/Walkway & force plate ==
  fp_dp : Inport
  fp_ie : Inport  Port=2
  FP Contact : Subsystem
  Force Plate : Subsystem
  Ground Contact : Subsystem
  Simulink-PS Converter3 : nesl_utility/Simulink-PS Converter  PhysicalDomain=network_engine_domain  SubClassName=ps_input  LeftPortType=input  RightPortType=output  PseudoPeriodic=off  Frequencies=[]  NoiseDistribution=none  NoiseParameters=[]  Unit=1  AffineConversion=off  InputFiltering=on  SimscapeFilterOrder=2  InputFilterTimeConstant=0.001  UdotUserProvided=1
  Simulink-PS Converter7 : nesl_utility/Simulink-PS Converter  PhysicalDomain=network_engine_domain  SubClassName=ps_input  LeftPortType=input  RightPortType=output  PseudoPeriodic=off  Frequencies=[]  NoiseDistribution=none  NoiseParameters=[]  Unit=1  AffineConversion=off  InputFiltering=on  SimscapeFilterOrder=2  InputFilterTimeConstant=0.0001  UdotUserProvided=1
  Transform2 : sm_lib/Frames and Transforms/Rigid Transform  TranslationMethod=StandardAxis  TranslationLengthUnit=m  TranslationStandardAxis=+Y  TranslationStandardOffset=0.1517  TranslationCartesianOffset=[0 0 0]  TranslationROffset=0  TranslationROffsetUnits=m  TranslationZOffset=0  TranslationZOffsetUnits=m  TranslationThetaOffset=0  TranslationThetaOffsetUnits=deg  RotationMethod=StandardAxis  RotationAngleUnits=deg  RotationStandardAxis=+X  RotationAngle=-90  RotationArbitraryAxis=[0 0 1]  FollAlignAxisA=+X  BaseAlignAxisA=+Y  FollAlignAxisB=+Y  BaseAlignAxisB=+Z  RotationSequenceAxes=FollowerAxes  RotationSequence=XYX  RotationSequenceAngles=[0 0 0]  RotationSequenceAnglesUnits=deg  RotationMatrix=[1 0 0; 0 1 0; 0 0 1]
  walkway_1_RIGID : Subsystem
  world : PMIOPort  Port=1  Side=Left
  foot surface : PMIOPort  Port=2  Side=Right
  fp_force : Outport
  fp_torque : Outport  Port=2
  grn_tor : Outport  Port=3
  fp_tor : Outport  Port=4
  wires:
  fp_dp/1 -> Simulink-PS Converter3/1
  fp_ie/1 -> Simulink-PS Converter7/1
  Force Plate/1(fp_force) -> fp_force/1
  Force Plate/2(fp_torque) -> fp_torque/1
  Ground Contact/1(grn_tor) -> grn_tor/1
  FP Contact/1(fp_tor) -> fp_tor/1
  connections:
  Force Plate/RConn1 -- FP Contact/RConn1
  FP Contact/LConn1 -- Ground Contact/LConn1 -- foot surface/RConn1
  Ground Contact/RConn1 -- Transform2/RConn1
  Simulink-PS Converter3/RConn1 -- Force Plate/LConn2
  Force Plate/LConn3 -- Simulink-PS Converter7/RConn1
  Transform2/LConn1 -- walkway_1_RIGID/LConn1 -- Force Plate/LConn1 -- world/RConn1

== system sim_impcont/Gait Emulator/Y Control ==
  inv_kin_y : Inport
  ground force : Inport  Port=2
  Y pos fdbk : Inport  Port=3
  Constant : Constant  Value=0
  PID Controller2 : simulink/Continuous/PID Controller  Controller=PID  TimeDomain=Continuous-time  SampleTime=-1  IntegratorMethod=Forward Euler  FilterMethod=Forward Euler  Form=Parallel  UseFilter=on  ControllerParametersSource=internal  P=80427.9807844241  I=313423.000955269  D=5118.61107289721  N=8615.608198692  InitialConditionSource=internal  InitialConditionForIntegrator=0  InitialConditionForFilter=0  ExternalReset=none  LimitOutput=on  UpperSaturationLimit=2*75*9.81  LowerSaturationLimit=-2*75*9.81  LinearizeAsGain=on  AntiWindupMode=clamping  Kb=1  TrackingMode=off  Kt=1  PParamMin=[]  PParamMax=[]  IParamMin=[]  IParamMax=[]  DParamMin=[]  DParamMax=[]  NParamMin=[]  NParamMax=[]  KbParamMin=[]  KbParamMax=[]  KtParamMin=[]  KtParamMax=[]  POutMin=[]  POutMax=[]  IOutMin=[]  IOutMax=[]  DOutMin=[]  DOutMax=[]  NOutMin=[]  NOutMax=[]  KbOutMin=[]  KbOutMax=[]  KtOutMin=[]  KtOutMax=[]  IntegratorOutMin=[]  IntegratorOutMax=[]  FilterOutMin=[]  FilterOutMax=[]  SumOutMin=[]  SumOutMax=[]  SumI1OutMin=[]  SumI1OutMax=[]  SumI2OutMin=[]  SumI2OutMax=[]  SumI3OutMin=[]  SumI3OutMax=[]  SumDOutMin=[]  SumDOutMax=[]  SaturationOutMin=[]  SaturationOutMax=[]  IntegratorContinuousStateAttributes=''  IntegratorStateMustResolveToSignalObject=off  IntegratorRTWStateStorageClass=Auto  FilterContinuousStateAttributes=''  FilterStateMustResolveToSignalObject=off  FilterRTWStateStorageClass=Auto  DifferentiatorICPrevScaledInput=0  DifferentiatorOutMin=[]  DifferentiatorOutMax=[]
  Sum3 : Sum  Inputs=|+-
  Switch1 : Switch  Criteria=u2 > Threshold  Threshold=5
  Y for : Outport
  wires:
  Y pos fdbk/1 -> Sum3/2
  Constant/1 -> Switch1/1
  Sum3/1 -> PID Controller2/1
  PID Controller2/1 -> Switch1/3
  inv_kin_y/1 -> Sum3/1
  Switch1/1 -> Y for/1
  ground force/1 -> Switch1/2

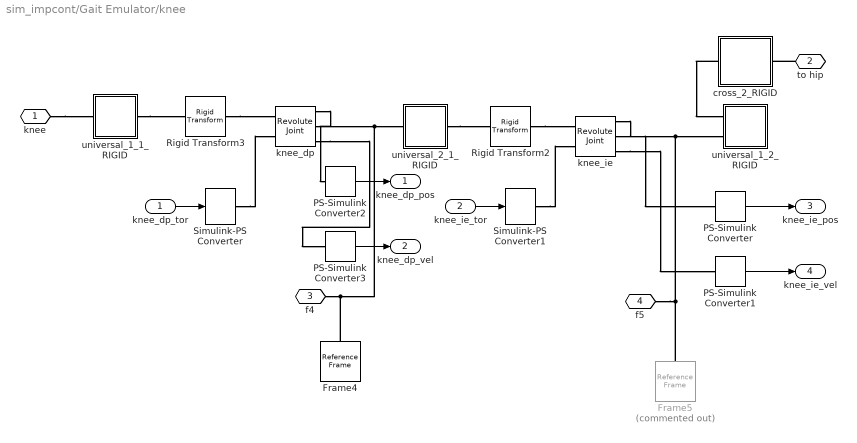
== system sim_impcont/Gait Emulator/knee  ==
  knee_dp_tor : Inport
  knee_ie_tor : Inport  Port=2
  Frame4 : sm_lib/Frames and Transforms/Reference Frame
  Frame5 : sm_lib/Frames and Transforms/Reference Frame  Commented=on
  PS-Simulink Converter{,1..3} (4 alike) : nesl_utility/PS-Simulink Converter  PhysicalDomain=network_engine_domain  SubClassName=ps_output  LeftPortType=input  RightPortType=output  PseudoPeriodic=off  Frequencies=[]  Unit=1  AffineConversion=off
  Rigid Transform2 : sm_lib/Frames and Transforms/Rigid Transform  TranslationMethod=None  TranslationLengthUnit=m  TranslationStandardAxis=+Z  TranslationStandardOffset=0  TranslationCartesianOffset=[0 0 0]  TranslationROffset=0  TranslationROffsetUnits=m  TranslationZOffset=0  TranslationZOffsetUnits=m  TranslationThetaOffset=0  TranslationThetaOffsetUnits=deg  RotationMethod=StandardAxis  RotationAngleUnits=deg  RotationStandardAxis=+Z  RotationAngle=-90  RotationArbitraryAxis=[0 0 1]  FollAlignAxisA=+X  BaseAlignAxisA=+Y  FollAlignAxisB=+Y  BaseAlignAxisB=+Z  RotationSequenceAxes=FollowerAxes  RotationSequence=XYX  RotationSequenceAngles=[0 0 0]  RotationSequenceAnglesUnits=deg  RotationMatrix=[1 0 0; 0 1 0; 0 0 1]
  Rigid Transform3 : sm_lib/Frames and Transforms/Rigid Transform  TranslationMethod=StandardAxis  TranslationLengthUnit=m  TranslationStandardAxis=+Z  TranslationStandardOffset=-0.034  TranslationCartesianOffset=[0 0 0]  TranslationROffset=0  TranslationROffsetUnits=m  TranslationZOffset=0  TranslationZOffsetUnits=m  TranslationThetaOffset=0  TranslationThetaOffsetUnits=deg  RotationMethod=StandardAxis  RotationAngleUnits=deg  RotationStandardAxis=+Y  RotationAngle=180  RotationArbitraryAxis=[0 0 1]  FollAlignAxisA=+X  BaseAlignAxisA=+Y  FollAlignAxisB=+Y  BaseAlignAxisB=+Z  RotationSequenceAxes=FollowerAxes  RotationSequence=XYX  RotationSequenceAngles=[0 0 0]  RotationSequenceAnglesUnits=deg  RotationMatrix=[1 0 0; 0 1 0; 0 0 1]
  Simulink-PS Converter : nesl_utility/Simulink-PS Converter  PhysicalDomain=network_engine_domain  SubClassName=ps_input  LeftPortType=input  RightPortType=output  PseudoPeriodic=off  Frequencies=[]  NoiseDistribution=none  NoiseParameters=[]  Unit=1  AffineConversion=off  InputFiltering=on  SimscapeFilterOrder=2  InputFilterTimeConstant=0.001  UdotUserProvided=1
  Simulink-PS Converter1 : nesl_utility/Simulink-PS Converter  PhysicalDomain=network_engine_domain  SubClassName=ps_input  LeftPortType=input  RightPortType=output  PseudoPeriodic=off  Frequencies=[]  NoiseDistribution=none  NoiseParameters=[]  Unit=1  AffineConversion=off  InputFiltering=on  SimscapeFilterOrder=2  InputFilterTimeConstant=0.001  UdotUserProvided=1
  cross_2_RIGID : Subsystem
  knee_dp : sm_lib/Joints/Revolute Joint  SenseConstraintForce=off  SenseConstraintForceX=off  SenseConstraintForceY=off  SenseConstraintForceZ=off  SenseConstraintTorque=off  SenseConstraintTorqueX=off  SenseConstraintTorqueY=off  SenseConstraintTorqueZ=off  SenseTotalForce=off  SenseTotalForceX=off  SenseTotalForceY=off  SenseTotalForceZ=off  SenseTotalTorque=off  SenseTotalTorqueX=off  SenseTotalTorqueY=off  SenseTotalTorqueZ=off  CompositeWrenchDir=FollowerOnBase  CompositeWrenchFrame=BaseFrame  EquilibriumPosition=0  EquilibriumPositionUnits=rad  SpringStiffness=stiff  SpringStiffnessUnits=m*N/rad  DampingCoefficient=damp  DampingCoefficientUnits=m*s*N/rad  TorqueActuationMode=InputTorque  MotionActuationMode=ComputedMotion  SensePosition=on  SenseVelocity=on  SenseAcceleration=off  SenseTorqueForce=off  PositionTargetSpecify=off  PositionTargetPriority=Low  PositionTargetValue=179.9999999999999999  PositionTargetValueUnits=deg  VelocityTargetSpecify=off  VelocityTargetPriority=High  VelocityTargetValue=0  VelocityTargetValueUnits=deg/s
  knee_ie : sm_lib/Joints/Revolute Joint  SenseConstraintForce=off  SenseConstraintForceX=off  SenseConstraintForceY=off  SenseConstraintForceZ=off  SenseConstraintTorque=off  SenseConstraintTorqueX=off  SenseConstraintTorqueY=off  SenseConstraintTorqueZ=off  SenseTotalForce=off  SenseTotalForceX=off  SenseTotalForceY=off  SenseTotalForceZ=off  SenseTotalTorque=off  SenseTotalTorqueX=off  SenseTotalTorqueY=off  SenseTotalTorqueZ=off  CompositeWrenchDir=FollowerOnBase  CompositeWrenchFrame=BaseFrame  EquilibriumPosition=0  EquilibriumPositionUnits=rad  SpringStiffness=stiff  SpringStiffnessUnits=m*N/rad  DampingCoefficient=damp  DampingCoefficientUnits=m*s*N/rad  TorqueActuationMode=InputTorque  MotionActuationMode=ComputedMotion  SensePosition=on  SenseVelocity=on  SenseAcceleration=off  SenseTorqueForce=off  PositionTargetSpecify=off  PositionTargetPriority=Low  PositionTargetValue=90  PositionTargetValueUnits=deg  VelocityTargetSpecify=off  VelocityTargetPriority=High  VelocityTargetValue=0  VelocityTargetValueUnits=deg/s
  universal_1_1_RIGID : Subsystem
  universal_1_2_RIGID : Subsystem
  universal_2_1_RIGID : Subsystem
  knee : PMIOPort  Port=1  Side=Right
  to hip : PMIOPort  Port=2  Side=Right
  f4 : PMIOPort  Port=3  Side=Left
  f5 : PMIOPort  Port=4  Side=Right
  knee_dp_pos : Outport
  knee_dp_vel : Outport  Port=2
  knee_ie_pos : Outport  Port=3
  knee_ie_vel : Outport  Port=4
  wires:
  knee_dp_tor/1 -> Simulink-PS Converter/1
  knee_ie_tor/1 -> Simulink-PS Converter1/1
  PS-Simulink Converter2/1 -> knee_dp_pos/1
  PS-Simulink Converter3/1 -> knee_dp_vel/1
  PS-Simulink Converter/1 -> knee_ie_pos/1
  PS-Simulink Converter1/1 -> knee_ie_vel/1
  connections:
  universal_1_1_RIGID/RConn1 -- Rigid Transform3/LConn1
  Rigid Transform3/RConn1 -- knee_dp/LConn1
  knee_dp/RConn1 -- f4/RConn1 -- Frame4/RConn1 -- universal_2_1_RIGID/LConn1
  Rigid Transform2/RConn1 -- knee_ie/LConn1
  knee_ie/RConn1 -- Frame5/RConn1 -- f5/RConn1 -- universal_1_2_RIGID/LConn2
  universal_2_1_RIGID/RConn1 -- Rigid Transform2/LConn1
  cross_2_RIGID/LConn1 -- universal_1_2_RIGID/LConn1
  to hip/RConn1 -- cross_2_RIGID/RConn1
  knee/RConn1 -- universal_1_1_RIGID/LConn1
  Simulink-PS Converter1/RConn1 -- knee_ie/LConn2
  Simulink-PS Converter/RConn1 -- knee_dp/LConn2
  knee_dp/RConn2 -- PS-Simulink Converter2/LConn1
  knee_dp/RConn3 -- PS-Simulink Converter3/LConn1
  knee_ie/RConn2 -- PS-Simulink Converter/LConn1
  knee_ie/RConn3 -- PS-Simulink Converter1/LConn1

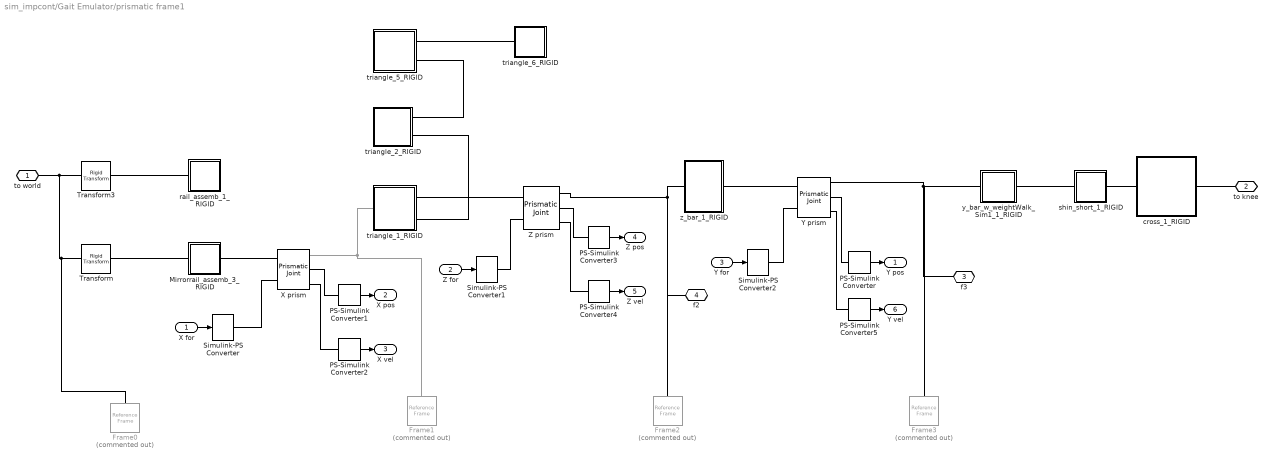
== system sim_impcont/Gait Emulator/prismatic frame1 ==
  X for : Inport
  Z for : Inport  Port=2
  Y for : Inport  Port=3
  Frame{0..3} (4 alike) : sm_lib/Frames and Transforms/Reference Frame  Commented=on
  Mirrorrail_assemb_3_RIGID : Subsystem
  PS-Simulink Converter{,1..5} (6 alike) : nesl_utility/PS-Simulink Converter  PhysicalDomain=network_engine_domain  SubClassName=ps_output  LeftPortType=input  RightPortType=output  PseudoPeriodic=off  Frequencies=[]  Unit=1  AffineConversion=off
  Simulink-PS Converter : nesl_utility/Simulink-PS Converter  PhysicalDomain=network_engine_domain  SubClassName=ps_input  LeftPortType=input  RightPortType=output  PseudoPeriodic=off  Frequencies=[]  NoiseDistribution=none  NoiseParameters=[]  Unit=1  AffineConversion=off  InputFiltering=on  SimscapeFilterOrder=2  InputFilterTimeConstant=0.001  UdotUserProvided=1
  Simulink-PS Converter1 : nesl_utility/Simulink-PS Converter  PhysicalDomain=network_engine_domain  SubClassName=ps_input  LeftPortType=input  RightPortType=output  PseudoPeriodic=off  Frequencies=[]  NoiseDistribution=none  NoiseParameters=[]  Unit=1  AffineConversion=off  InputFiltering=on  SimscapeFilterOrder=2  InputFilterTimeConstant=0.001  UdotUserProvided=1
  Simulink-PS Converter2 : nesl_utility/Simulink-PS Converter  PhysicalDomain=network_engine_domain  SubClassName=ps_input  LeftPortType=input  RightPortType=output  PseudoPeriodic=off  Frequencies=[]  NoiseDistribution=none  NoiseParameters=[]  Unit=1  AffineConversion=off  InputFiltering=on  SimscapeFilterOrder=2  InputFilterTimeConstant=0.001  UdotUserProvided=1
  Transform : sm_lib/Frames and Transforms/Rigid Transform  TranslationMethod=Cartesian  TranslationLengthUnit=m  TranslationStandardAxis=+Z  TranslationStandardOffset=0  TranslationCartesianOffset=[3.2000000000000011 1.4389401389271192 0.54097612726828137]  TranslationROffset=0  TranslationROffsetUnits=m  TranslationZOffset=0  TranslationZOffsetUnits=m  TranslationThetaOffset=0  TranslationThetaOffsetUnits=deg  RotationMethod=None  RotationAngleUnits=deg  RotationStandardAxis=+Z  RotationAngle=0.0  RotationArbitraryAxis=[0 0 1]  FollAlignAxisA=+X  BaseAlignAxisA=+Y  FollAlignAxisB=+Y  BaseAlignAxisB=+Z  RotationSequenceAxes=FollowerAxes  RotationSequence=XYX  RotationSequenceAngles=[0 0 0]  RotationSequenceAnglesUnits=deg  RotationMatrix=[1 0 0; 0 1 0; 0 0 1]
  Transform3 : sm_lib/Frames and Transforms/Rigid Transform  TranslationMethod=Cartesian  TranslationLengthUnit=m  TranslationStandardAxis=+Z  TranslationStandardOffset=0  TranslationCartesianOffset=[3.2000000000000011 1.4389401389271192 -0.54097612726828137]  TranslationROffset=0  TranslationROffsetUnits=m  TranslationZOffset=0  TranslationZOffsetUnits=m  TranslationThetaOffset=0  TranslationThetaOffsetUnits=deg  RotationMethod=None  RotationAngleUnits=deg  RotationStandardAxis=+Z  RotationAngle=0.0  RotationArbitraryAxis=[0 0 1]  FollAlignAxisA=+X  BaseAlignAxisA=+Y  FollAlignAxisB=+Y  BaseAlignAxisB=+Z  RotationSequenceAxes=FollowerAxes  RotationSequence=XYX  RotationSequenceAngles=[0 0 0]  RotationSequenceAnglesUnits=deg  RotationMatrix=[1 0 0; 0 1 0; 0 0 1]
  X prism : sm_lib/Joints/Prismatic Joint  SenseConstraintForce=off  SenseConstraintForceX=off  SenseConstraintForceY=off  SenseConstraintForceZ=off  SenseConstraintTorque=off  SenseConstraintTorqueX=off  SenseConstraintTorqueY=off  SenseConstraintTorqueZ=off  SenseTotalForce=off  SenseTotalForceX=off  SenseTotalForceY=off  SenseTotalForceZ=off  SenseTotalTorque=off  SenseTotalTorqueX=off  SenseTotalTorqueY=off  SenseTotalTorqueZ=off  CompositeWrenchDir=FollowerOnBase  CompositeWrenchFrame=BaseFrame  EquilibriumPosition=0  EquilibriumPositionUnits=m  SpringStiffness=stiff  SpringStiffnessUnits=N/m  DampingCoefficient=damp  DampingCoefficientUnits=s*N/m  TorqueActuationMode=InputTorque  MotionActuationMode=ComputedMotion  SensePosition=on  SenseVelocity=on  SenseAcceleration=off  SenseTorqueForce=off  PositionTargetSpecify=off  PositionTargetPriority=Low  PositionTargetValue=-3.2  PositionTargetValueUnits=m  VelocityTargetSpecify=off  VelocityTargetPriority=High  VelocityTargetValue=0  VelocityTargetValueUnits=m/s
  Y prism : sm_lib/Joints/Prismatic Joint  SenseConstraintForce=off  SenseConstraintForceX=off  SenseConstraintForceY=off  SenseConstraintForceZ=off  SenseConstraintTorque=off  SenseConstraintTorqueX=off  SenseConstraintTorqueY=off  SenseConstraintTorqueZ=off  SenseTotalForce=off  SenseTotalForceX=off  SenseTotalForceY=off  SenseTotalForceZ=off  SenseTotalTorque=off  SenseTotalTorqueX=off  SenseTotalTorqueY=off  SenseTotalTorqueZ=off  CompositeWrenchDir=FollowerOnBase  CompositeWrenchFrame=BaseFrame  EquilibriumPosition=0  EquilibriumPositionUnits=m  SpringStiffness=stiff  SpringStiffnessUnits=N/m  DampingCoefficient=damp  DampingCoefficientUnits=s*N/m  TorqueActuationMode=InputTorque  MotionActuationMode=ComputedMotion  SensePosition=on  SenseVelocity=on  SenseAcceleration=off  SenseTorqueForce=off  PositionTargetSpecify=off  PositionTargetPriority=Low  PositionTargetValue=-0.1  PositionTargetValueUnits=m  VelocityTargetSpecify=off  VelocityTargetPriority=High  VelocityTargetValue=0  VelocityTargetValueUnits=m/s
  Z prism : sm_lib/Joints/Prismatic Joint  SenseConstraintForce=off  SenseConstraintForceX=off  SenseConstraintForceY=off  SenseConstraintForceZ=off  SenseConstraintTorque=off  SenseConstraintTorqueX=off  SenseConstraintTorqueY=off  SenseConstraintTorqueZ=off  SenseTotalForce=off  SenseTotalForceX=off  SenseTotalForceY=off  SenseTotalForceZ=off  SenseTotalTorque=off  SenseTotalTorqueX=off  SenseTotalTorqueY=off  SenseTotalTorqueZ=off  CompositeWrenchDir=FollowerOnBase  CompositeWrenchFrame=BaseFrame  EquilibriumPosition=0  EquilibriumPositionUnits=m  SpringStiffness=stiff  SpringStiffnessUnits=N/m  DampingCoefficient=damp  DampingCoefficientUnits=s*N/m  TorqueActuationMode=InputTorque  MotionActuationMode=ComputedMotion  SensePosition=on  SenseVelocity=on  SenseAcceleration=off  SenseTorqueForce=off  PositionTargetSpecify=on  PositionTargetPriority=Low  PositionTargetValue=0  PositionTargetValueUnits=m  VelocityTargetSpecify=off  VelocityTargetPriority=High  VelocityTargetValue=0  VelocityTargetValueUnits=m/s
  cross_1_RIGID : Subsystem
  rail_assemb_1_RIGID : Subsystem
  shin_short_1_RIGID : Subsystem
  triangle_1_RIGID : Subsystem
  triangle_2_RIGID : Subsystem
  triangle_5_RIGID : Subsystem
  triangle_6_RIGID : Subsystem
  y_bar_w_weightWalk_Sim1_1_RIGID : Subsystem
  z_bar_1_RIGID : Subsystem
  to world : PMIOPort  Port=1  Side=Left
  to knee : PMIOPort  Port=2  Side=Right
  f3 : PMIOPort  Port=3  Side=Left
  f2 : PMIOPort  Port=4  Side=Right
  Y pos : Outport
  X pos : Outport  Port=2
  X vel : Outport  Port=3
  Z pos : Outport  Port=4
  Z vel : Outport  Port=5
  Y vel : Outport  Port=6
  wires:
  X for/1 -> Simulink-PS Converter/1
  Z for/1 -> Simulink-PS Converter1/1
  Y for/1 -> Simulink-PS Converter2/1
  PS-Simulink Converter/1 -> Y pos/1
  PS-Simulink Converter1/1 -> X pos/1
  PS-Simulink Converter2/1 -> X vel/1
  PS-Simulink Converter3/1 -> Z pos/1
  PS-Simulink Converter4/1 -> Z vel/1
  PS-Simulink Converter5/1 -> Y vel/1
  connections:
  cross_1_RIGID/RConn1 -- to knee/RConn1
  to world/RConn1 -- Frame0/RConn1 -- Transform/LConn1 -- Transform3/LConn1
  Frame1/RConn1 -- X prism/RConn1 -- triangle_1_RIGID/LConn1
  Z prism/LConn1 -- triangle_1_RIGID/RConn1
  Mirrorrail_assemb_3_RIGID/RConn1 -- X prism/LConn1
  Y prism/LConn1 -- z_bar_1_RIGID/RConn1
  Z prism/RConn1 -- Frame2/RConn1 -- f2/RConn1 -- z_bar_1_RIGID/LConn1
  Y prism/RConn1 -- Frame3/RConn1 -- f3/RConn1 -- y_bar_w_weightWalk_Sim1_1_RIGID/LConn1
  shin_short_1_RIGID/RConn1 -- cross_1_RIGID/LConn1
  shin_short_1_RIGID/LConn1 -- y_bar_w_weightWalk_Sim1_1_RIGID/RConn1
  triangle_2_RIGID/RConn2 -- triangle_1_RIGID/RConn2
  triangle_6_RIGID/RConn1 -- triangle_5_RIGID/RConn1
  triangle_2_RIGID/RConn1 -- triangle_5_RIGID/RConn2
  Simulink-PS Converter1/RConn1 -- Z prism/LConn2
  Simulink-PS Converter/RConn1 -- X prism/LConn2
  Simulink-PS Converter2/RConn1 -- Y prism/LConn2
  Y prism/RConn2 -- PS-Simulink Converter/LConn1
  Transform3/RConn1 -- rail_assemb_1_RIGID/LConn1
  Transform/RConn1 -- Mirrorrail_assemb_3_RIGID/LConn1
  PS-Simulink Converter5/LConn1 -- Y prism/RConn3
  Z prism/RConn2 -- PS-Simulink Converter3/LConn1
  Z prism/RConn3 -- PS-Simulink Converter4/LConn1
  X prism/RConn2 -- PS-Simulink Converter1/LConn1
  X prism/RConn3 -- PS-Simulink Converter2/LConn1
